simulink model "sgMdl_IO135_InterModuleSync_Loopback"  (R2024b)
settings: Solver=FixedStepAuto  StartTime=0.0  StopTime=inf  RelTol=1e-3  EnableMultiTasking=on
libraries: speedgoatlib_IO135 x6, speedgoatlib_interrupt x1
Description:
  | IO135 - Inter-Module Synchronization Loopback
settings Model: sg_rtwmakecfg_data=_sglibc_  ModifiedByFormat=Speedgoat  SimulationMode=external  ExtModeTrigDuration=100000  Creator=Speedgoat  LastModifiedBy=Speedgoat
settings SolverCC: ConcurrentTasks=on  AlgebraicLoopSolver=TrustRegion  PositivePriorityOrder=on  AutoInsertRateTranBlk=on  InsertRTBMode=Never (minimum delay)
settings DataIOCC: SaveFormat=StructureWithTime  ReturnWorkspaceOutputs=off
settings OptimizationCC: BlockReduction=off  OptimizeBlockIOStorage=off  BufferReuse=off  GlobalBufferReuse=off  ExpressionFolding=off  LocalBlockOutputs=off
settings DebuggingCC: TasksWithSamePriorityMsg=none  SFExecutionAtInitializationDiag=none  ArithmeticOperatorsInVariantConditions=warning
settings HardwareCC: ProdBitPerLong=64  ProdLongLongMode=on  ProdHWDeviceType=Intel->x86-64 (Linux 64)
settings ModelReferenceCC: EnableRefExpFcnMdlSchedulingChecks=on
settings SFSimCC: SimUseLocalCustomCode=off  CustomCodeUndefinedFunction=UseInterfaceOnly
settings RTWCC: Description=Speedgoat Real-Time Target Machine  SystemTargetFile=speedgoat.tlc  TemplateMakefile=slrealtime_default_tmf  PostCodeGenCommand=sg.model.build.makeCfg(bdroot, buildInfo);  RTWUseLocalCustomCode=off  Toolchain=Simulink Real-Time Toolchain  BuildConfiguration=Faster Runs  TargetLang=C++  GPUComputeCapability=3.5  DLArmComputeVersion=19.05
settings CodeAppCC: StateflowObjectComments=on
settings SimulinkRealTimeTargetCC: SubcomponentCodeInterfacePackaging=Reusable function  InstructionSetFMA=off  LogToMDFFile=off  SLRTFileLogMaxRuns=10  UseGCCFastMath=on
settings ConfigComp: CovBoundaryAbsTol=1.0e-5

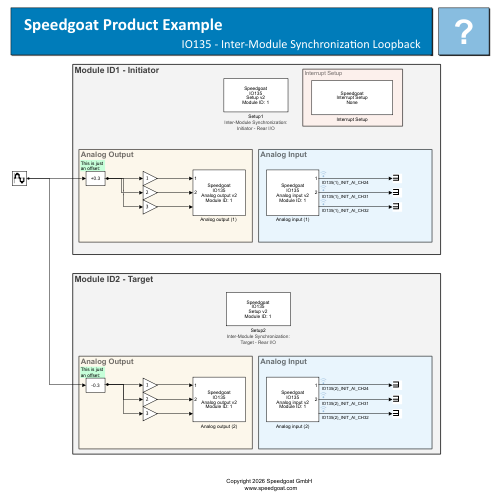
[thumbnail: Simulink's stored preview of the top-level diagram]
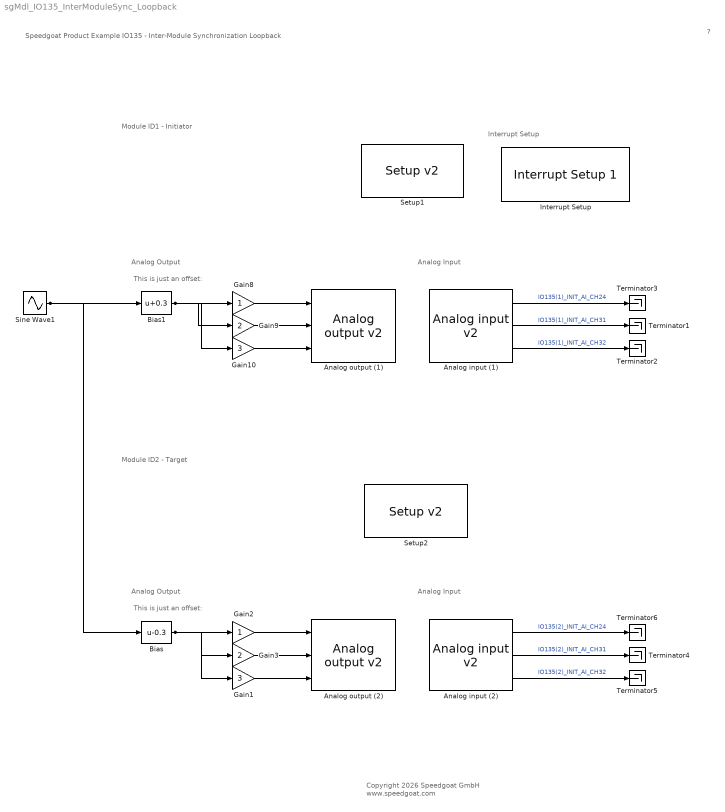
== system sgMdl_IO135_InterModuleSync_Loopback ==
  note: This is just an offset:
  note: Analog Input
  note: Analog Output
  note: Analog Input
  note: Analog Output
  note: Module ID1 - Initiator
  note: Interrupt Setup
  note: Module ID2 - Target
  note: This is just an offset:
  note: Speedgoat Product Example
      | IO135 - Inter-Module Synchronization Loopback
  note: ?
  note: Copyright 2026 Speedgoat GmbH
      |  www.speedgoat.com
  Analog input (1) : speedgoatlib_IO135/Analog input v2   parModuleId=1  parSampleTime=-1  parPciSlot=-1  parAdcChannels=[24 31 32]  parAdcVoltageRange=[2 2 2 2]  parAdcOversamplRate=[1 1 1 1]  parAdcContSampling=0  parAdcDmaEnable=1  parAdcActiveDmaDevices=[1 1 1 1]  parAdcFrameSize=10
      settings: SourceProductName=Simulink Real-Time: Speedgoat I/O Driver Library
  Analog input (2) : speedgoatlib_IO135/Analog input v2   parModuleId=2  parSampleTime=-1  parPciSlot=-1  parAdcChannels=[24 31 32]  parAdcVoltageRange=[2 2 2 2]  parAdcOversamplRate=[1 1 1 1]  parAdcContSampling=0  parAdcDmaEnable=1  parAdcActiveDmaDevices=[1 1 1 1]  parAdcFrameSize=10
      settings: SourceProductName=Simulink Real-Time: Speedgoat I/O Driver Library
  "Analog output (1) " : speedgoatlib_IO135/Analog output v2   parModuleId=1  parSampleTime=-1  parPciSlot=-1  parDacChannels=[1 2 9]  parDacVoltageRange=[5 5 5 5 5 5 5 5 5 5 5 5 5 5 5 5]  parDacInitValues=[0 0 0]  parDacReset=[1 1 1]  parDacSyncOut=1  parDacDmaEnable=1  parDacActiveDmaDevices=[1 1 1 1]  parDacDmaLatency=2  parDacFrameSize=1
      settings: SourceProductName=Simulink Real-Time: Speedgoat I/O Driver Library
  Analog output (2) : speedgoatlib_IO135/Analog output v2   parModuleId=2  parSampleTime=-1  parPciSlot=-1  parDacChannels=[1 2 9]  parDacVoltageRange=[5 5 5 5 5 5 5 5 5 5 5 5 5 5 5 5]  parDacInitValues=[0 0 0]  parDacReset=[1 1 1]  parDacSyncOut=1  parDacDmaEnable=1  parDacActiveDmaDevices=[1 1 1 1]  parDacDmaLatency=2  parDacFrameSize=1
      settings: SourceProductName=Simulink Real-Time: Speedgoat I/O Driver Library
  Bias : Bias  Bias=-0.3  SaturateOnIntegerOverflow=off
  Bias1 : Bias  Bias=0.3  SaturateOnIntegerOverflow=off
  Gain1 : Gain  Gain=3
  Gain10 : Gain  Gain=3
  Gain2 : Gain
  Gain3 : Gain  Gain=2
  Gain8 : Gain
  Gain9 : Gain  Gain=2
  Interrupt Setup : speedgoatlib_interrupt/Interrupt Setup 1  parModuleTrigger=on  parPollingMode=off  parPriorityConf=High  parPriority=241  confStartFcn=IO135_start_public  confStopFcn=IO135_stop_public  confIsrFcn=IO135_isr_public  confMapFcn=IO135_map_public  confHookFile=io135_int_hooks.c  confIrqNr=-1  confIsPolling=off  confModID=16776961  confSelectedInt=Speedgoat IO135 DMA interrupt  confSelectedId=1  confSelectedChannel=[]  confData=[]  confForcePollingMode=off
  Setup1 : speedgoatlib_IO135/Setup v2   parPciSlot=-1  parModuleId=1  parInterModuleSync=Initiator - Rear I/O  parConvClockBaseRate=20MHz  parConvClock1Divider=clockDivider  parConvClock2Divider=2000  parFrameTriggerEnable=on  parFrameTriggerDivider=frameSize  parConvClock1BaseRate=1  parConvClock2BaseRate=1  parFrameTriggerClock=1  parAdcChannels=[24,31,32]  parAdcRange1=+-10V  parAdcRange2=+-10V  parAdcRange3=+-10V  parAdcRange4=+-10V  parAdcVoltageRange=[2 2 2 2]  parAdcOversampling1=None  parAdcOversampling2=None  parAdcOversampling3=None  parAdcOversampling4=None  parAdcOversamplRate=[1 1 1 1]  parAdcContSampling=off  parAdcDataCorrection=Automatic  parAdcCorrectionActive={}  parAdcCorrectionPm5V={'1','0','0';'2','0','0';'3','0','0';'4','0','0';'5','0','0';'6','0','0';'7','0','0';'8','0','0';'9','0','0';'10','0','0';'11','0','0';'12','0','0';'13','0','0';'14','0',' 0';'15','0','0';'16','0','0';'17','0','0';'18','0','0';'19','0','0';'20','0','0';'21','0','0';'22','0','0';'23','0','0';'24','0','0';'25','0','0';'26','0','0';'27','0','0';'28','0','0';'29','0','0';'30','0','0';'31','0','0';'32','0','0'}  parAdcCorrectionPm10V={'1','0','0';'2','0','0';'3','0','0';'4','0','0';'5','0','0';'6','0','0';'7','0','0';'8','0','0';'9','0','0';'10','0','0';'11','0','0';'12','0','0';'13','0','0';'14','0',' 0';'15','0','0';'16','0','0';'17','0','0';'18','0','0';'19','0','0';'20','0','0';'21','0','0';'22','0','0';'23','0','0';'24','0','0';'25','0','0';'26','0','0';'27','0','0';'28','0','0';'29','0','0';'30','0','0';'31','0','0';'32','0','0'}  parAdcDmaEnable=on  parAdcDmaClock=Clock 1  parAdcFrameSize_=frameSize  parAdcSampleTime_=-1  parAdcActiveDmaDevices=[1 1 1 1]  parAdcFrameTriggerEnable=1  parAdcFrameSize=10  parAdcSampleTime=0.001  parDacChannels=[1,2,9]  parDacInitValues=0  parDacReset=1  parDacRange1=+-10V  parDacRange2=+-10V  parDacRange3=+-10V  parDacRange4=+-10V  parDacRange5=+-10V  parDacRange6=+-10V  parDacRange7=+-10V  parDacRange8=+-10V  parDacRange9=+-10V  parDacRange10=+-10V  parDacRange11=+-10V  parDacRange12=+-10V  parDacRange13=+-10V  parDacRange14=+-10V  parDacRange15=+-10V  parDacRange16=+-10V  parDacVoltageRange=[5 5 5 5 5 5 5 5 5 5 5 5 5 5 5 5]  parDacSyncOut=on  parDacDataCorrection=Automatic  parDacCorrectionActive={}  parDacCorrection5V={'1','0','0';'2','0','0';'3','0','0';'4','0','0';'5','0','0';'6','0','0';'7','0','0';'8','0','0';'9','0','0';'10','0','0';'11','0','0';'12','0','0';'13','0','0';'14','0',' 0';'15','0','0';'16','0','0'}  parDacCorrection10V={'1','0','0';'2','0','0';'3','0','0';'4','0','0';'5','0','0';'6','0','0';'7','0','0';'8','0','0';'9','0','0';'10','0','0';'11','0','0';'12','0','0';'13','0','0';'14','0',' 0';'15','0','0';'16','0','0'}  parDacCorrection10_8V={'1','0','0';'2','0','0';'3','0','0';'4','0','0';'5','0','0';'6','0','0';'7','0','0';'8','0','0';'9','0','0';'10','0','0';'11','0','0';'12','0','0';'13','0','0';'14','0',' 0';'15','0','0';'16','0','0'}  parDacCorrectionPm5V={'1','0','0';'2','0','0';'3','0','0';'4','0','0';'5','0','0';'6','0','0';'7','0','0';'8','0','0';'9','0','0';'10','0','0';'11','0','0';'12','0','0';'13','0','0';'14','0',' 0';'15','0','0';'16','0','0'}  parDacCorrectionPm10V={'1','0','0';'2','0','0';'3','0','0';'4','0','0';'5','0','0';'6','0','0';'7','0','0';'8','0','0';'9','0','0';'10','0','0';'11','0','0';'12','0','0';'13','0','0';'14','0',' 0';'15','0','0';'16','0','0'}  parDacCorrectionPm10_8V={'1','0','0';'2','0','0';'3','0','0';'4','0','0';'5','0','0';'6','0','0';'7','0','0';'8','0','0';'9','0','0';'10','0','0';'11','0','0';'12','0','0';'13','0','0';'14','0',' 0';'15','0','0';'16','0','0'}  parDacDmaEnable=on  parDacDmaLatency=Until next frame  parDacDmaClock=Clock 1  parDacFrameSize_=1  parDacSampleTime_=-1  parDacActiveDmaDevices=[1 1 1 1]  parDacFrameTriggerEnable=1  parDacFrameSize=1  parDacSampleTime=0.0001  parDoChannels=1  parDoInitValues=0  parDoReset=1  parDiChannels=5  parDiDebounceEnable=off  parDiDebounceTime=0  parDiDebounceValue=0  parDioPullRefFront=Pull-up 3.3V  parDioPullRefRear=Floating
      settings: SourceProductName=Simulink Real-Time: Speedgoat I/O Driver Library
      settings: AttributesFormatString=|
      | Inter-Module Synchronization:
      | %<parInterModuleSync>
  Setup2 : speedgoatlib_IO135/Setup v2   parPciSlot=-1  parModuleId=2  parInterModuleSync=Target - Rear I/O  parConvClockBaseRate=20MHz  parConvClock1Divider=clockDivider  parConvClock2Divider=2000  parFrameTriggerEnable=on  parFrameTriggerDivider=frameSize  parConvClock1BaseRate=1  parConvClock2BaseRate=1  parFrameTriggerClock=1  parAdcChannels=[24,31,32]  parAdcRange1=+-10V  parAdcRange2=+-10V  parAdcRange3=+-10V  parAdcRange4=+-10V  parAdcVoltageRange=[2 2 2 2]  parAdcOversampling1=None  parAdcOversampling2=None  parAdcOversampling3=None  parAdcOversampling4=None  parAdcOversamplRate=[1 1 1 1]  parAdcContSampling=off  parAdcDataCorrection=Automatic  parAdcCorrectionActive={}  parAdcCorrectionPm5V={'1','0','0';'2','0','0';'3','0','0';'4','0','0';'5','0','0';'6','0','0';'7','0','0';'8','0','0';'9','0','0';'10','0','0';'11','0','0';'12','0','0';'13','0','0';'14','0',' 0';'15','0','0';'16','0','0';'17','0','0';'18','0','0';'19','0','0';'20','0','0';'21','0','0';'22','0','0';'23','0','0';'24','0','0';'25','0','0';'26','0','0';'27','0','0';'28','0','0';'29','0','0';'30','0','0';'31','0','0';'32','0','0'}  parAdcCorrectionPm10V={'1','0','0';'2','0','0';'3','0','0';'4','0','0';'5','0','0';'6','0','0';'7','0','0';'8','0','0';'9','0','0';'10','0','0';'11','0','0';'12','0','0';'13','0','0';'14','0',' 0';'15','0','0';'16','0','0';'17','0','0';'18','0','0';'19','0','0';'20','0','0';'21','0','0';'22','0','0';'23','0','0';'24','0','0';'25','0','0';'26','0','0';'27','0','0';'28','0','0';'29','0','0';'30','0','0';'31','0','0';'32','0','0'}  parAdcDmaEnable=on  parAdcDmaClock=Clock 1  parAdcFrameSize_=frameSize  parAdcSampleTime_=-1  parAdcActiveDmaDevices=[1 1 1 1]  parAdcFrameTriggerEnable=1  parAdcFrameSize=10  parAdcSampleTime=0.001  parDacChannels=[1,2,9]  parDacInitValues=0  parDacReset=1  parDacRange1=+-10V  parDacRange2=+-10V  parDacRange3=+-10V  parDacRange4=+-10V  parDacRange5=+-10V  parDacRange6=+-10V  parDacRange7=+-10V  parDacRange8=+-10V  parDacRange9=+-10V  parDacRange10=+-10V  parDacRange11=+-10V  parDacRange12=+-10V  parDacRange13=+-10V  parDacRange14=+-10V  parDacRange15=+-10V  parDacRange16=+-10V  parDacVoltageRange=[5 5 5 5 5 5 5 5 5 5 5 5 5 5 5 5]  parDacSyncOut=on  parDacDataCorrection=Automatic  parDacCorrectionActive={}  parDacCorrection5V={'1','0','0';'2','0','0';'3','0','0';'4','0','0';'5','0','0';'6','0','0';'7','0','0';'8','0','0';'9','0','0';'10','0','0';'11','0','0';'12','0','0';'13','0','0';'14','0',' 0';'15','0','0';'16','0','0'}  parDacCorrection10V={'1','0','0';'2','0','0';'3','0','0';'4','0','0';'5','0','0';'6','0','0';'7','0','0';'8','0','0';'9','0','0';'10','0','0';'11','0','0';'12','0','0';'13','0','0';'14','0',' 0';'15','0','0';'16','0','0'}  parDacCorrection10_8V={'1','0','0';'2','0','0';'3','0','0';'4','0','0';'5','0','0';'6','0','0';'7','0','0';'8','0','0';'9','0','0';'10','0','0';'11','0','0';'12','0','0';'13','0','0';'14','0',' 0';'15','0','0';'16','0','0'}  parDacCorrectionPm5V={'1','0','0';'2','0','0';'3','0','0';'4','0','0';'5','0','0';'6','0','0';'7','0','0';'8','0','0';'9','0','0';'10','0','0';'11','0','0';'12','0','0';'13','0','0';'14','0',' 0';'15','0','0';'16','0','0'}  parDacCorrectionPm10V={'1','0','0';'2','0','0';'3','0','0';'4','0','0';'5','0','0';'6','0','0';'7','0','0';'8','0','0';'9','0','0';'10','0','0';'11','0','0';'12','0','0';'13','0','0';'14','0',' 0';'15','0','0';'16','0','0'}  parDacCorrectionPm10_8V={'1','0','0';'2','0','0';'3','0','0';'4','0','0';'5','0','0';'6','0','0';'7','0','0';'8','0','0';'9','0','0';'10','0','0';'11','0','0';'12','0','0';'13','0','0';'14','0',' 0';'15','0','0';'16','0','0'}  parDacDmaEnable=on  parDacDmaLatency=Until next frame  parDacDmaClock=Clock 1  parDacFrameSize_=1  parDacSampleTime_=-1  parDacActiveDmaDevices=[1 1 1 1]  parDacFrameTriggerEnable=1  parDacFrameSize=1  parDacSampleTime=0.0001  parDoChannels=1  parDoInitValues=0  parDoReset=1  parDiChannels=5  parDiDebounceEnable=off  parDiDebounceTime=0  parDiDebounceValue=0  parDioPullRefFront=Pull-up 3.3V  parDioPullRefRear=Floating
      settings: SourceProductName=Simulink Real-Time: Speedgoat I/O Driver Library
      settings: AttributesFormatString=|
      | Inter-Module Synchronization:
      | %<parInterModuleSync>
  Sine Wave1 : Sin  Amplitude=0.3  Frequency=50  SampleTime=0.001
  Terminator{1..6} (6 alike) : Terminator
  wires:
  Sine Wave1/1 -> Bias/1, Bias1/1
  Analog input (2)/2 -> Terminator4/1  "IO135(2)_INIT_AI_CH31"
  Gain2/1 -> Analog output (2)/1
  Gain3/1 -> Analog output (2)/2
  Gain1/1 -> Analog output (2)/3
  Analog input (1)/3 -> Terminator2/1  "IO135(1)_INIT_AI_CH32"
  Analog input (1)/2 -> Terminator1/1  "IO135(1)_INIT_AI_CH31"
  Gain9/1 -> "Analog output (1) "/2
  Analog input (2)/1 -> Terminator6/1  "IO135(2)_INIT_AI_CH24"
  Gain10/1 -> "Analog output (1) "/3
  Analog input (2)/3 -> Terminator5/1  "IO135(2)_INIT_AI_CH32"
  Gain8/1 -> "Analog output (1) "/1
  Analog input (1)/1 -> Terminator3/1  "IO135(1)_INIT_AI_CH24"
  Bias/1 -> Gain2/1, Gain1/1, Gain3/1
  Bias1/1 -> Gain8/1, Gain10/1, Gain9/1
